simulink model "CM475A_TSG31CfgAndUse"  (R2013b)
settings: Solver=FixedStepDiscrete  SolverMode=SingleTasking  StartTime=0.0  StopTime=0.5  FixedStep=0.00005  RelTol=1e-3
undefined symbols (not defined in the file): ELECGLBPRM_PWMPERDMIN_NANOSEC_U32, sigbuilder_block, SysSt1, TSG31CfgAndUseAdcStrtOfCnvn2Offs, TSG31CfgAndUseAdcStrtOfCnvnMotCtrlPeakOffs, TSG31CfgAndUseAdcStrtOfCnvnMotCtrlVlyOffs, TSG31CfgAndUseMtrAg0SPIStart, TSG31CfgAndUsePwmDbnd, TSG31UPD_NANOSEC_U32
libraries: simulink x11, CM475A_TSG31CfgAndUse_ModelLibrary_Rev001 x11
(part 1 of 4)
settings Model: Creator=nz3zln  LastModifiedBy=nz3zln
settings SolverCC: AutoInsertRateTranBlk=on  InsertRTBMode=Always
settings DataIOCC: LimitDataPoints=off  SaveFormat=Structure  ReturnWorkspaceOutputs=on
settings OptimizationCC: BlockReduction=off  InlineParams=on  ZeroExternalMemoryAtStartup=off  ZeroInternalMemoryAtStartup=off  OptimizeModelRefInitCode=on  LifeSpan=1
settings DebuggingCC: SignalInfNanChecking=error  SignalRangeChecking=warning  UnderspecifiedInitializationDetection=Simplified  SolverPrmCheckMsg=error  InheritedTsInSrcMsg=error  DiscreteInheritContinuousMsg=error  SingleTaskRateTransMsg=error  TasksWithSamePriorityMsg=error  SigSpecEnsureSampleTimeMsg=error  CheckMatrixSingularityMsg=error  ParameterUnderflowMsg=error  ParameterPrecisionLossMsg=error  ParameterTunabilityLossMsg=error  FixptConstUnderflowMsg=warning  FixptConstOverflowMsg=warning  VectorMatrixConversionMsg=error  SignalLabelMismatchMsg=error  UnconnectedInputMsg=error  UnconnectedOutputMsg=error  UnconnectedLineMsg=error  SFcnCompatibilityMsg=error  UniqueDataStoreMsg=warning  BusObjectLabelMismatch=error  RootOutportRequireBusObject=error  AssertControl=DisableAll  ModelReferenceIOMsg=error  ModelReferenceVersionMismatchMessage=warning  ModelReferenceIOMismatchMessage=error  ModelReferenceCSMismatchMessage=warning  ModelReferenceDataLoggingMessage=error  StateNameClashWarn=warning  StrictBusMsg=ErrorOnBusTreatedAsVector  NonBusSignalsTreatedAsBus=error  SFUnexpectedBacktrackingDiag=error  SFInvalidInputDataAccessInChartInitDiag=error  SFNoUnconditionalDefaultTransitionDiag=error  SFTransitionOutsideNaturalParentDiag=error  SFUnconditionalTransitionShadowingDiag=error  SFUndirectedBroadcastEventsDiag=error
settings ModelReferenceCC: ModelReferenceNumInstancesAllowed=Single
settings RTWCC: SystemTargetFile=autosar.tlc  GenCodeOnly=on  TemplateMakefile=ert_default_tmf  Description=AUTOSAR  GenerateReport=on  ProcessScript=autosar_make_rtw_hook  LaunchReport=on
settings CodeAppCC: GenerateComments=off  IgnoreCustomStorageClasses=off  CustomSymbolStrType=$N$R$M  CustomSymbolStrBlkIO=$N$M  SimulinkBlockComments=off
settings STFCustomTargetCC: ParMdlRefBuildCompliant=on  CompOptLevelCompliant=on  IncludeMdlTerminateFcn=off  CombineOutputUpdateFcns=on  SuppressErrorStatus=on  ERTFirstTimeCompliant=on  ERTCustomFileBanners=on  SupportNonFinite=off  SupportComplex=off  SupportContinuousTime=off  SupportNonInlinedSFcns=off  MATLABClassNameForMDSCustomization=Simulink.SoftwareTarget.ERTCustomization  AutosarCompliant=on  GRTInterface=off  SystemTargetFile=autosar.tlc
settings ERTTargetCC: CodeReplacementLibrary=ANSI_C  ConcurrentExecutionCompliant=off  IncludeMdlTerminateFcn=off  SuppressErrorStatus=on  SupportNonFinite=off  SupportComplex=off  ModelStepFunctionPrototypeControlCompliant=off  CPPClassGenCompliant=off  AutosarCompliant=on  InlinedParameterPlacement=NonHierarchical  ERTCustomFileTemplate=example_file_process.tlc  EnableUserReplacementTypes=on

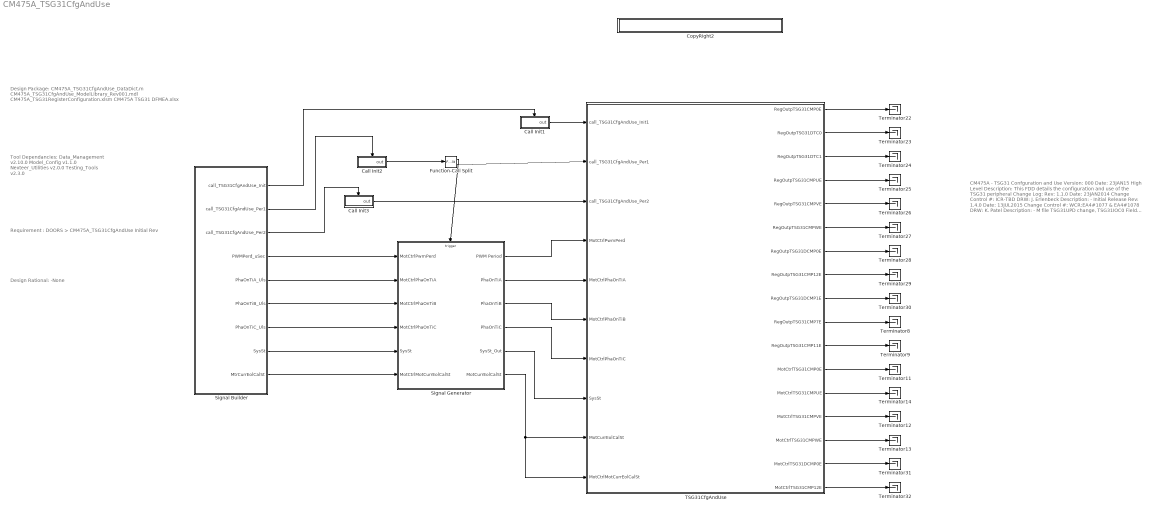
== system CM475A_TSG31CfgAndUse ==
  note: CM475A - TSG31 Confguration and Use
      |
      | Version: 000
      | Date: 23JAN15
      |
      | High Level Description:
      | This FDD details the configuration and use of the TSG31 peripheral
      |
      | Change Log:
      |
      | Rev: 1.1.0
      | Date: 23JAN2014
      | Change Control #: ICR-TBD
      | DRW: J. Erlenbeck
      | Description:
      | - Initial Release
      |
      | Rev: 1.4.0
      | Date: 13JUL2015
      | Change Control #: WCR:EA4#1077 & EA4#1078
      | DRW: K. Patel
      | Description:
      | - M file TSG31UPD change, TSG31IOC0 Field value change in excel
      |
      | Rev: 1.5.0
      | Date: 08SEP2016
      | Change Control #: WCR:EA4#7447
      | DRW: G. McCann
      | Description:
      | - M file init values changed:
      | 	MotCtrlTSG31DCMP0E
      | 	MotCtrlTSG31CMP0E
      | 	MotCtrlTSG31CMP12E
      | 	MotCtrlTSG31CMPWE
      | 	MotCtrlTSG31CMPVE
      | 	MotCtrlTSG31CMPUE
      |
      | Rev: 1.6.0
      | Date: 27SEP2016
      | Change Control #: WCR:EA4#7447
      | DRW: J. Erlenbeck
      | Description:
      | - Removed symbolic outputs, updated to newer modeling standards
      |   without changing any code functionality.
  note: Tool Dependancies:
      |
      | Data_Management v2.10.0
      | Model_Config v1.1.0
      | Nexteer_Utilities v2.0.0
      | Testing_Tools v2.3.0
  note: Design Package:
      |
      | CM475A_TSG31CfgAndUse_DataDict.m
      | CM475A_TSG31CfgAndUse_ModelLibrary_Rev001.mdl
      | CM475A_TSG31RegisterConfiguration.xlsm
      | CM475A TSG31 DFMEA.xlsx
  note: Requirement :
      |
      | DOORS > CM475A_TSG31CfgAndUse Initial Rev
  note: Design Rational:
      |
      | -None
  Call Init1 : Subsystem  TreatAsAtomicUnit=on
  Call Init2 : Subsystem  TreatAsAtomicUnit=on
  Call Init3 : Subsystem  RequirementInfo="{}  %GIDa_2aef89e2_413b_41a9_8abb_59aacf2ea464"  TreatAsAtomicUnit=on
  CopyRight2 : Subsystem  Description=|  mask(Copyright Information){none=on}
      | Copyright info block.                                               
      |                                                                     
      | Place copyright information at the top of every subsystem in design.
      mask prompts: none "No parameters"
      mask help: Place copyright information at the top of every subsystem in design.
      mask Display:
      | NxtrConf = 'Nexteer Confidential';
      | 
      | sys = bdroot; %handle for the current model ("system")
      | first = get_param(sys,'Created');
      | first = first(end-3:end);  %year is last four digits
      | 
      | last = get_param(sys,'LastModifiedDate');
      | if isempty(last)
      |     last = datestr(now,'yyyy');
      | else
      |     last = last(end-3:end);
      | end
      | 
      | if strcmp(first,last)
      |     fprintf('%s -- Copyright %s Nexteer',NxtrConf,first)
      | else
      |     fprintf('%s -- %s%s- %s Nexteer',NxtrConf,char(169),first,last)
      | end
  Function-Call Split : FunctionCallSplit
  Signal Builder : Subsystem  Tag=STV Subsys  RequirementInfo={} %GIDa_2822100e_29fa_4197_9ccc_01864625f252  LoadFcn=sigbuilder_block('load');  StartFcn=sigbuilder_block('start');  StopFcn=sigbuilder_block('stop');  ClipboardFcn=sigbuilder_block('clipboard');  mask(Sigbuilder block){}
      mask help: Simulink:masks:SigbuilderBlock_MD
      mask init:
      | if ~strcmp(get_param(bdroot(gcbh),'SimulationStatus'),'stopped') tuvar = sigbuilder_block('maskInit'); end
      settings: CopyFcn=sigbuilder_block('copy');  DeleteFcn=sigbuilder_block('delete');  ModelCloseFcn=sigbuilder_block('modelClose');  PreSaveFcn=sigbuilder_block('preSave');  PauseFcn=sigbuilder_block('pause');  ContinueFcn=sigbuilder_block('continue');  NameChangeFcn=sigbuilder_block('namechange');  OpenFcn=sigbuilder_block('open',[94.9655 670.345 1191.72 616.966 ]);  CloseFcn=sigbuilder_block('close');
      mask Display: plot(0, 0, 100, 100,[2, 2, 32, 32, 2], [68, 8, 8, 68, 68],[32, 2], [38, 38], [32, 19, 2],[53, 60, 44], [32, 17, 17, 2],[16, 16, 31, 31]);txt = getActiveGroup(gcbh);text(2, 100, txt,'verticalAlignment', 'top');
  Signal Generator : Subsystem  TreatAsAtomicUnit=on
  TSG31CfgAndUse : Subsystem
  Terminator{8..9,11..14,22..32} (17 alike) : Terminator
  wires:
  Call Init2/1(out) -> Function-Call Split/1
  Call Init3/1(out) -> TSG31CfgAndUse/3(call_TSG31CfgAndUse_Per2)
  Call Init1/1(out) -> TSG31CfgAndUse/1(call_TSG31CfgAndUse_Init1)
  Signal Builder/3(call_TSG31CfgAndUse_Per2) -> Call Init3/Enable
  Signal Builder/2(call_TSG31CfgAndUse_Per1) -> Call Init2/Enable
  Signal Builder/1(call_TSG31CfgAndUse_Init) -> Call Init1/Enable
  TSG31CfgAndUse/1(RegOutpTSG31CMP0E) -> Terminator22/1
  TSG31CfgAndUse/2(RegOutpTSG31DTC0) -> Terminator23/1
  TSG31CfgAndUse/3(RegOutpTSG31DTC1) -> Terminator24/1
  TSG31CfgAndUse/4(RegOutpTSG31CMPUE) -> Terminator25/1
  TSG31CfgAndUse/5(RegOutpTSG31CMPVE) -> Terminator26/1
  TSG31CfgAndUse/6(RegOutpTSG31CMPWE) -> Terminator27/1
  TSG31CfgAndUse/7(RegOutpTSG31DCMP0E) -> Terminator28/1
  TSG31CfgAndUse/8(RegOutpTSG31CMP12E) -> Terminator29/1
  TSG31CfgAndUse/9(RegOutpTSG31DCMP1E) -> Terminator30/1
  TSG31CfgAndUse/10(RegOutpTSG31CMP7E) -> Terminator8/1
  TSG31CfgAndUse/11(RegOutpTSG31CMP11E) -> Terminator9/1
  TSG31CfgAndUse/12(MotCtrlTSG31CMP0E) -> Terminator11/1
  TSG31CfgAndUse/13(MotCtrlTSG31CMPUE) -> Terminator14/1
  TSG31CfgAndUse/14(MotCtrlTSG31CMPVE) -> Terminator12/1
  TSG31CfgAndUse/15(MotCtrlTSG31CMPWE) -> Terminator13/1
  TSG31CfgAndUse/16(MotCtrlTSG31DCMP0E) -> Terminator31/1
  TSG31CfgAndUse/17(MotCtrlTSG31CMP12E) -> Terminator32/1
  Function-Call Split/1 -> Signal Generator/Trigger
  Function-Call Split/2 -> TSG31CfgAndUse/2(call_TSG31CfgAndUse_Per1)
  Signal Builder/7(PhaOnTiC_Uls) -> Signal Generator/4(MotCtrlPhaOnTiC)
  Signal Builder/8(SysSt) -> Signal Generator/5(SysSt)
  Signal Builder/6(PhaOnTiB_Uls) -> Signal Generator/3(MotCtrlPhaOnTiB)
  Signal Builder/5(PhaOnTiA_Uls) -> Signal Generator/2(MotCtrlPhaOnTiA)
  Signal Builder/9(MtrCurrEolCalSt) -> Signal Generator/6(MotCtrlMotCurrEolCalSt)
  Signal Builder/4(PWMPerd_uSec) -> Signal Generator/1(MotCtrlPwmPerd)
  Signal Generator/3(PhaOnTiB) -> TSG31CfgAndUse/6(MotCtrlPhaOnTiB)
  Signal Generator/2(PhaOnTiA) -> TSG31CfgAndUse/5(MotCtrlPhaOnTiA)
  Signal Generator/1(PWM Period) -> TSG31CfgAndUse/4(MotCtrlPwmPerd)
  Signal Generator/4(PhaOnTiC) -> TSG31CfgAndUse/7(MotCtrlPhaOnTiC)
  Signal Generator/5(SysSt_Out) -> TSG31CfgAndUse/8(SysSt)
  Signal Generator/6(MotCurrEolCalSt) -> TSG31CfgAndUse/10(MotCtrlMotCurrEolCalSt), TSG31CfgAndUse/9(MotCurrEolCalSt)

== system CM475A_TSG31CfgAndUse/Call Init1 ==
  Enable : EnablePort
  Function Call Trigger : simulink/Ports & Subsystems/Function-Call Generator  RequirementInfo={} %GIDa_ff755a2e_49d1_45f7_8591_3ce0ef475338  sample_time=0.002  numberOfIterations=1
  out : Outport
  wires:
  Function Call Trigger/1 -> out/1

== system CM475A_TSG31CfgAndUse/Call Init2 ==
  Enable : EnablePort
  Function Call Trigger : simulink/Ports & Subsystems/Function-Call Generator  RequirementInfo={} %GIDa_286e4ac1_b4ae_4a31_a667_8384976eef74  sample_time=0.00005  numberOfIterations=1
  out : Outport
  wires:
  Function Call Trigger/1 -> out/1

== system CM475A_TSG31CfgAndUse/Call Init3 ==
  Enable : EnablePort
  Function Call Trigger : simulink/Ports & Subsystems/Function-Call Generator  RequirementInfo={} %GIDa_f9d17251_db1b_46c2_b3b0_280e370bf339  sample_time=0.002  numberOfIterations=1
  out : Outport
  wires:
  Function Call Trigger/1 -> out/1

== system CM475A_TSG31CfgAndUse/CopyRight2 ==

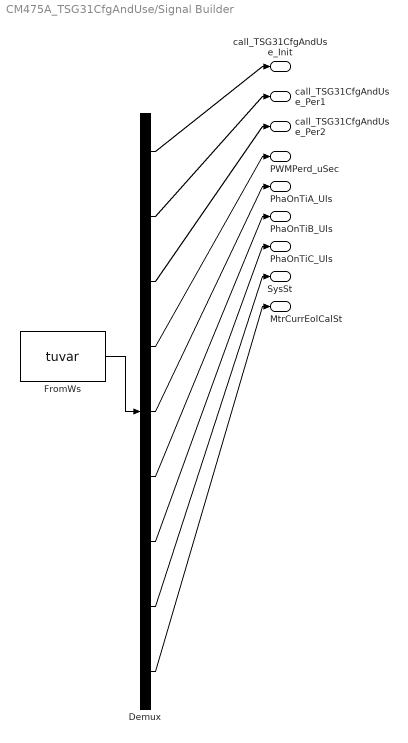
== system CM475A_TSG31CfgAndUse/Signal Builder ==
  Demux : Demux  Tag=STV Demux  Outputs=9
  FromWs : FromWorkspace  Tag=STV FromWs  VariableName=tuvar  SampleTime=0
      SigBuilderData=|
      | common.afterFinalStr = 'Extrapolate'
      | common.sampleTime = 0
      | dataSet(1).timeRange = [0 0.5]
      | dataSet(1).name = 'Group 1'
      | dataSet(2).timeRange = [0 0.5]
      | dataSet(2).name = 'Group 2'
      | dataSet(3).timeRange = [0 1.2]
      | dataSet(3).name = 'Group 3'
      | dataSet(4).timeRange = [0 5]
      | dataSet(4).name = 'Group 4'
      | dataSet(5).timeRange = [0 10]
      | dataSet(5).name = 'Group 5'
      | dataSet(6).timeRange = [0 8]
      | dataSet(6).name = 'Group 6'
      | sbobj.Groups(1).Name = 'Group 1'
      | sbobj.Groups(1).Signals(1).Name = 'call_TSG31CfgAndUse_Init'
      | sbobj.Groups(1).Signals(1).XData = [0 0.001 0.001 0.5]
      | sbobj.Groups(1).Signals(1).YData = [1 1 0 0]
      | sbobj.Groups(1).Signals(2).Name = 'call_TSG31CfgAndUse_Per1'
      | sbobj.Groups(1).Signals(2).XData = [0 0.002 0.002 0.5]
      | sbobj.Groups(1).Signals(2).YData = [0 0 1 1]
      | sbobj.Groups(1).Signals(3).Name = 'call_TSG31CfgAndUse_Per2'
      | sbobj.Groups(1).Signals(3).XData = [0 0.002 0.002 8]
      | sbobj.Groups(1).Signals(3).YData = [0 0 1 1]
      | sbobj.Groups(1).Signals(4).Name = 'PWMPerd_uSec'
      | sbobj.Groups(1).Signals(4).XData = [0 0.5]
      | sbobj.Groups(1).Signals(4).YData = [50 50]
      | sbobj.Groups(1).Signals(5).Name = 'PhaOnTiA_Uls'
      | sbobj.Groups(1).Signals(5).XData = [0 0.0102040816327 0.0204081632653 0.030612244898 0.0408163265306 0.0510204081633 0.0612244897959 0.0714285714286 0.0816326530612 0.0918367346939 0.102040816327 0.112244897959 0.122448979592 0.132653061224 0.142857142857 0.15306122449 0.163265306122 0.173469387755 0.183673469388 0.19387755102 0.204081632653 0.214285714286 0.224489795918 0.234693877551 0.244897959184 0.255102040816 0.265306122449 0.275510204082 0.285714285714 0.295918367347 0.30612244898 0.316326530612 0.326530612245 0.336734693878 0.34693877551 0.357142857143 0.367346938776 0.377551020408 0.387755102041 0.397959183673 0.408163265306 0.418367346939 0.428571428571 0.438775510204 0.448979591837 0.459183673469 0.469387755102 0.479591836735 0.489795918367 0.5]
      | sbobj.Groups(1).Signals(5).YData = [0.5 0.563938580842 0.626827291955 0.68763350244 0.745358776002 0.799055265246 0.847841275302 0.890915741234 0.927571381503 0.957206311508 0.979333926518 0.993590891707 0.9997431081 0.997689556475 0.987463956091 0.969234211025 0.943299653187 0.910086127298 0.870138998538 0.824114197654 0.772767450605 0.716941869559 0.657554109012 0.595579314351 0.53203510999 0.46796489001 0.404420685649 0.342445890988 0.283058130441 0.227232549395 0.175885802346 0.129861001462 0.0899138727015 0.0567003468135 0.0307657889751 0.0125360439091 0.0023104435254 0.000256891899656 0.00640910829277 0.0206660734817 0.0427936884921 0.0724286184973 0.109084258766 0.152158724698 0.200944734754 0.254641223998 0.31236649756 0.373172708045 0.436061419158 0.5]
      | sbobj.Groups(1).Signals(6).Name = 'PhaOnTiB_Uls'
      | sbobj.Groups(1).Signals(6).XData = [0 0.1 0.1 0.2 0.2 0.3 0.3 0.4 0.4 0.5]
      | sbobj.Groups(1).Signals(6).YData = [1 1 0 0 1 1 0 0 1 1]
      | sbobj.Groups(1).Signals(7).Name = 'PhaOnTiC_Uls'
      | sbobj.Groups(1).Signals(7).XData = [0 0.125 0.125 0.25 0.25 0.375 0.375 0.5]
      | sbobj.Groups(1).Signals(7).YData = [0 1 0 1 0 1 0 1]
      | sbobj.Groups(1).Signals(8).Name = 'SysSt'
      | sbobj.Groups(1).Signals(8).XData = [0 0 0.5 0.5 1 1 1.5 1.5 2 2 2.5 2.5 3 3 3.5 3.5 4 4 4.5 4.5 5 5 5.5 5.5 6 6 6.5 6.5 7 7 7.5 7.5 8 8]
      | sbobj.Groups(1).Signals(8).YData = [0 2 2 0 0 2 2 0 0 2 2 0 0 2 2 0 0 2 2 0 0 2 2 0 0 2 2 0 0 2 2 0 0 2]
      | sbobj.Groups(1).Signals(9).Name = 'MtrCurrEolCalSt'
      | sbobj.Groups(1).Signals(9).XData = [0 0.5 1 1 1.5 1.5 2 2 2.5 2.5 3 3 3.5 3.5 4 4 4.5 4.5 5 5 5.5 5.5 6 6 6.5 6.5 7 7 7.5 7.5 8]
      | sbobj.Groups(1).Signals(9).YData = [0 0 0 2 2 0 0 2 2 0 0 2 2 0 0 2 2 0 0 2 2 0 0 2 2 0 0 2 2 0 0]
      | sbobj.Groups(1).TimeRange = [0 0.5]
      | sbobj.Groups(2).Name = 'Group 2'
      | sbobj.Groups(2).Signals(1).Name = 'call_TSG31CfgAndUse_Init'
      | sbobj.Groups(2).Signals(1).XData = [0 0.001 0.001 0.5]
      | sbobj.Groups(2).Signals(1).YData = [1 1 0 0]
      | sbobj.Groups(2).Signals(2).Name = 'call_TSG31CfgAndUse_Per1'
      | sbobj.Groups(2).Signals(2).XData = [0 0.002 0.002 0.5]
      | sbobj.Groups(2).Signals(2).YData = [0 0 1 1]
      | sbobj.Groups(2).Signals(3).Name = 'call_TSG31CfgAndUse_Per2'
      | sbobj.Groups(2).Signals(3).XData = [0 0.002 0.002 8]
      | sbobj.Groups(2).Signals(3).YData = [0 0 1 1]
      | sbobj.Groups(2).Signals(4).Name = 'PWMPerd_uSec'
      | sbobj.Groups(2).Signals(4).XData = [0 0.5]
      | sbobj.Groups(2).Signals(4).YData = [0 0]
      | sbobj.Groups(2).Signals(5).Name = 'PhaOnTiA_Uls'
      | sbobj.Groups(2).Signals(5).XData = [0 0.5]
      | sbobj.Groups(2).Signals(5).YData = [4 4]
      | sbobj.Groups(2).Signals(6).Name = 'PhaOnTiB_Uls'
      | sbobj.Groups(2).Signals(6).XData = [0 0.2 0.2 0.5]
      | sbobj.Groups(2).Signals(6).YData = [0 0 5 5]
      | sbobj.Groups(2).Signals(7).Name = 'PhaOnTiC_Uls'
      | sbobj.Groups(2).Signals(7).XData = [0 0.5]
      | sbobj.Groups(2).Signals(7).YData = [0 0]
      | sbobj.Groups(2).Signals(8).Name = 'SysSt'
      | sbobj.Groups(2).Signals(8).XData = [0 0 0.5 0.5 1 1 1.5 1.5 2 2 2.5 2.5 3 3 3.5 3.5 4 4 4.5 4.5 5 5 5.5 5.5 6 6 6.5 6.5 7 7 7.5 7.5 8 8]
      | sbobj.Groups(2).Signals(8).YData = [0 2 2 0 0 2 2 0 0 2 2 0 0 2 2 0 0 2 2 0 0 2 2 0 0 2 2 0 0 2 2 0 0 2]
      | sbobj.Groups(2).Signals(9).Name = 'MtrCurrEolCalSt'
      | sbobj.Groups(2).Signals(9).XData = [0 0 0.5 0.5 1 1 1.5 1.5 2 2 2.5 2.5 3 3 3.5 3.5 4 4 4.5 4.5 5 5 5.5 5.5 6 6 6.5 6.5 7 7 7.5 7.5 8 8]
      | sbobj.Groups(2).Signals(9).YData = [0 2 2 0 0 2 2 0 0 2 2 0 0 2 2 0 0 2 2 0 0 2 2 0 0 2 2 0 0 2 2 0 0 2]
      | sbobj.Groups(2).TimeRange = [0 0.5]
      | sbobj.Groups(3).Name = 'Group 3'
      | sbobj.Groups(3).Signals(1).Name = 'call_TSG31CfgAndUse_Init'
      | sbobj.Groups(3).Signals(1).XData = [0 0.001 0.001 1.2]
      | sbobj.Groups(3).Signals(1).YData = [1 1 0 0]
      | sbobj.Groups(3).Signals(2).Name = 'call_TSG31CfgAndUse_Per1'
      | sbobj.Groups(3).Signals(2).XData = [0 0.002 0.002 1.2]
      | sbobj.Groups(3).Signals(2).YData = [0 0 1 1]
      | sbobj.Groups(3).Signals(3).Name = 'call_TSG31CfgAndUse_Per2'
      | sbobj.Groups(3).Signals(3).XData = [0 0.002 0.002 8]
      | sbobj.Groups(3).Signals(3).YData = [0 0 1 1]
      | sbobj.Groups(3).Signals(4).Name = 'PWMPerd_uSec'
      | sbobj.Groups(3).Signals(4).XData = [0 1.2]
      | sbobj.Groups(3).Signals(4).YData = [0 0]
      | sbobj.Groups(3).Signals(5).Name = 'PhaOnTiA_Uls'
      | sbobj.Groups(3).Signals(5).XData = [0 1 1 1.2]
      | sbobj.Groups(3).Signals(5).YData = [0 0 -5 -5]
      | sbobj.Groups(3).Signals(6).Name = 'PhaOnTiB_Uls'
      | sbobj.Groups(3).Signals(6).XData = [0 1.2]
      | sbobj.Groups(3).Signals(6).YData = [0.5 0.5]
      | sbobj.Groups(3).Signals(7).Name = 'PhaOnTiC_Uls'
      | sbobj.Groups(3).Signals(7).XData = [0 1.2]
      | sbobj.Groups(3).Signals(7).YData = [0 0]
      | sbobj.Groups(3).Signals(8).Name = 'SysSt'
      | sbobj.Groups(3).Signals(8).XData = [0 0 0.5 0.5 1 1 1.5 1.5 2 2 2.5 2.5 3 3 3.5 3.5 4 4 4.5 4.5 5 5 5.5 5.5 6 6 6.5 6.5 7 7 7.5 7.5 8 8]
      | sbobj.Groups(3).Signals(8).YData = [0 2 2 0 0 2 2 0 0 2 2 0 0 2 2 0 0 2 2 0 0 2 2 0 0 2 2 0 0 2 2 0 0 2]
      | sbobj.Groups(3).Signals(9).Name = 'MtrCurrEolCalSt'
      | sbobj.Groups(3).Signals(9).XData = [0 0 0.5 0.5 1 1 1.5 1.5 2 2 2.5 2.5 3 3 3.5 3.5 4 4 4.5 4.5 5 5 5.5 5.5 6 6 6.5 6.5 7 7 7.5 7.5 8 8]
      | sbobj.Groups(3).Signals(9).YData = [0 2 2 0 0 2 2 0 0 2 2 0 0 2 2 0 0 2 2 0 0 2 2 0 0 2 2 0 0 2 2 0 0 2]
      | sbobj.Groups(3).TimeRange = [0 1.2]
      | sbobj.Groups(4).Name = 'Group 4'
      | sbobj.Groups(4).Signals(1).Name = 'call_TSG31CfgAndUse_Init'
      | sbobj.Groups(4).Signals(1).XData = [0 0.001 0.001 5]
      | sbobj.Groups(4).Signals(1).YData = [1 1 0 0]
      | sbobj.Groups(4).Signals(2).Name = 'call_TSG31CfgAndUse_Per1'
      | sbobj.Groups(4).Signals(2).XData = [0 0.002 0.002 5]
      | sbobj.Groups(4).Signals(2).YData = [0 0 1 1]
      | sbobj.Groups(4).Signals(3).Name = 'call_TSG31CfgAndUse_Per2'
      | sbobj.Groups(4).Signals(3).XData = [0 0.002 0.002 8]
      | sbobj.Groups(4).Signals(3).YData = [0 0 1 1]
      | sbobj.Groups(4).Signals(4).Name = 'PWMPerd_uSec'
      | sbobj.Groups(4).Signals(4).XData = [0 5]
      | sbobj.Groups(4).Signals(4).YData = [0 0]
      | sbobj.Groups(4).Signals(5).Name = 'PhaOnTiA_Uls'
      | sbobj.Groups(4).Signals(5).XData = [0 1.5 2 5]
      | sbobj.Groups(4).Signals(5).YData = [0 1.35 0.6 -3]
      | sbobj.Groups(4).Signals(6).Name = 'PhaOnTiB_Uls'
      | sbobj.Groups(4).Signals(6).XData = [0 0.1 0.1 5]
      | sbobj.Groups(4).Signals(6).YData = [0 0 2 2]
      | sbobj.Groups(4).Signals(7).Name = 'PhaOnTiC_Uls'
      | sbobj.Groups(4).Signals(7).XData = [0 5]
      | sbobj.Groups(4).Signals(7).YData = [0 0]
      | sbobj.Groups(4).Signals(8).Name = 'SysSt'
      | sbobj.Groups(4).Signals(8).XData = [0 0 0.5 0.5 1 1 1.5 1.5 2 2 2.5 2.5 3 3 3.5 3.5 4 4 4.5 4.5 5 5 5.5 5.5 6 6 6.5 6.5 7 7 7.5 7.5 8 8]
      | sbobj.Groups(4).Signals(8).YData = [0 2 2 0 0 2 2 0 0 2 2 0 0 2 2 0 0 2 2 0 0 2 2 0 0 2 2 0 0 2 2 0 0 2]
      | sbobj.Groups(4).Signals(9).Name = 'MtrCurrEolCalSt'
      | sbobj.Groups(4).Signals(9).XData = [0 0 0.5 0.5 1 1 1.5 1.5 2 2 2.5 2.5 3 3 3.5 3.5 4 4 4.5 4.5 5 5 5.5 5.5 6 6 6.5 6.5 7 7 7.5 7.5 8 8]
      | sbobj.Groups(4).Signals(9).YData = [0 2 2 0 0 2 2 0 0 2 2 0 0 2 2 0 0 2 2 0 0 2 2 0 0 2 2 0 0 2 2 0 0 2]
      | sbobj.Groups(4).TimeRange = [0 5]
      | sbobj.Groups(5).Name = 'Group 5'
      | sbobj.Groups(5).Signals(1).Name = 'call_TSG31CfgAndUse_Init'
      | sbobj.Groups(5).Signals(1).XData = [0 0.001 0.001 10]
      | sbobj.Groups(5).Signals(1).YData = [1 1 0 0]
      | sbobj.Groups(5).Signals(2).Name = 'call_TSG31CfgAndUse_Per1'
      | sbobj.Groups(5).Signals(2).XData = [0 0.002 0.002 10]
      | sbobj.Groups(5).Signals(2).YData = [0 0 1 1]
      | sbobj.Groups(5).Signals(3).Name = 'call_TSG31CfgAndUse_Per2'
      | sbobj.Groups(5).Signals(3).XData = [0 0.002 0.002 10]
      | sbobj.Groups(5).Signals(3).YData = [0 0 1 1]
      | sbobj.Groups(5).Signals(4).Name = 'PWMPerd_uSec'
      | sbobj.Groups(5).Signals(4).XData = [0 10]
      | sbobj.Groups(5).Signals(4).YData = [0 0]
      | sbobj.Groups(5).Signals(5).Name = 'PhaOnTiA_Uls'
      | sbobj.Groups(5).Signals(5).XData = [0 10]
      | sbobj.Groups(5).Signals(5).YData = [2 2]
      | sbobj.Groups(5).Signals(6).Name = 'PhaOnTiB_Uls'
      | sbobj.Groups(5).Signals(6).XData = [0 10]
      | sbobj.Groups(5).Signals(6).YData = [2.5 2.5]
      | sbobj.Groups(5).Signals(7).Name = 'PhaOnTiC_Uls'
      | sbobj.Groups(5).Signals(7).XData = [0 4 5 10]
      | sbobj.Groups(5).Signals(7).YData = [0 59 70 511]
      | sbobj.Groups(5).Signals(8).Name = 'SysSt'
      | sbobj.Groups(5).Signals(8).XData = [0 0 0.5 0.5 1 1 1.5 1.5 2 2 2.5 2.5 3 3 3.5 3.5 4 4 4.5 4.5 5 5 5.5 5.5 6 6 6.5 6.5 7 7 7.5 7.5 8 8 10]
      | sbobj.Groups(5).Signals(8).YData = [0 2 2 0 0 2 2 0 0 2 2 0 0 2 2 0 0 2 2 0 0 2 2 0 0 2 2 0 0 2 2 0 0 2 2]
      | sbobj.Groups(5).Signals(9).Name = 'MtrCurrEolCalSt'
      | sbobj.Groups(5).Signals(9).XData = [0 0 0.5 0.5 1 1 1.5 1.5 2 2 2.5 2.5 3 3 3.5 3.5 4 4 4.5 4.5 5 5 5.5 5.5 6 6 6.5 6.5 7 7 7.5 7.5 8 8 10]
      | sbobj.Groups(5).Signals(9).YData = [0 2 2 0 0 2 2 0 0 2 2 0 0 2 2 0 0 2 2 0 0 2 2 0 0 2 2 0 0 2 2 0 0 2 2]
      | sbobj.Groups(6).Name = 'Group 6'
      | sbobj.Groups(6).Signals(1).Name = 'call_TSG31CfgAndUse_Init'
      | sbobj.Groups(6).Signals(1).XData = [0 0.001 0.001 8]
      | sbobj.Groups(6).Signals(1).YData = [1 1 0 0]
      | sbobj.Groups(6).Signals(2).Name = 'call_TSG31CfgAndUse_Per1'
      | sbobj.Groups(6).Signals(2).XData = [0 0.002 0.002 8]
      | sbobj.Groups(6).Signals(2).YData = [0 0 1 1]
      | sbobj.Groups(6).Signals(3).Name = 'call_TSG31CfgAndUse_Per2'
      | sbobj.Groups(6).Signals(3).XData = [0 0.002 0.002 8]
      | sbobj.Groups(6).Signals(3).YData = [0 0 1 1]
      | sbobj.Groups(6).Signals(4).Name = 'PWMPerd_uSec'
      | sbobj.Groups(6).Signals(4).XData = [0 0.125 0.25 0.375 0.5 0.625 0.75 0.875 1 1.125 1.25 1.375 1.5 1.625 1.75 1.875 2 2.125 2.25 2.375 2.5 2.625 2.75 2.875 3 3.125 3.25 3.375 3.5 3.625 3.75 3.875 4 4.125 4.25 4.375 4.5 4.625 4.75 4.875 5 5.125 5.25 5.375 5.5 5.625 5.75 5.875 6 6.125 6.25 6.375 6.5 6.625 6.75 6.875 7 7.125 7.25 7.375 7.5 7.625 7.75 7.875 8]
      | sbobj.Groups(6).Signals(4).YData = [1 1.70710678119 2 1.70710678119 1 0.292893218813 0 0.292893218813 1 1.70710678119 2 1.70710678119 1 0.292893218813 0 0.292893218813 1 1.70710678119 2 1.70710678119 1 0.292893218813 0 0.292893218813 1 1.70710678119 2 1.70710678119 1 0.292893218813 0 0.292893218813 1 1.70710678119 2 1.70710678119 1 0.292893218813 0 0.292893218813 1 1.70710678119 2 1.70710678119 1 0.292893218813 0 0.292893218813 1 1.70710678119 2 1.70710678119 1 0.292893218813 0 0.292893218813 1 1.70710678119 2 1.70710678119 1 0.292893218813 0 0.292893218813 1]
      | sbobj.Groups(6).Signals(5).Name = 'PhaOnTiA_Uls'
      | sbobj.Groups(6).Signals(5).XData = [0 0.5 0.5 1 1 1.5 1.5 2 2 2.5 2.5 3 3 3.5 3.5 4 4 4.5 5 5.5 6 6.5 6.5 7 7.5 7.5 8]
      | sbobj.Groups(6).Signals(5).YData = [10 10 -10 -10 10 10 -10 -10 10 10 -10 -10 7 5.5 -5 -5.5 0 0 0 0 0 0 -0.5 0 -0.5 0 0]
      | sbobj.Groups(6).Signals(6).Name = 'PhaOnTiB_Uls'
      | sbobj.Groups(6).Signals(6).XData = [0 1 1 2 2 3 3 4 4 5 5 6 6 7 7 8]
      | sbobj.Groups(6).Signals(6).YData = [8.8 8.8 -8.8 -8.8 8.8 8.8 -8.8 -8.8 8.8 8.8 -8.8 -8.8 8.8 8.8 -8.8 -8.6]
      | sbobj.Groups(6).Signals(7).Name = 'PhaOnTiC_Uls'
      | sbobj.Groups(6).Signals(7).XData = [0 8]
      | sbobj.Groups(6).Signals(7).YData = [70 70]
      | sbobj.Groups(6).Signals(8).Name = 'SysSt'
      | sbobj.Groups(6).Signals(8).XData = [0 0.5 0.5 1 1 1.5 1.5 2 2 2.5 2.5 3 3 3.5 3.5 4 4 4.5 4.5 5 5 5.5 5.5 6 6 6.5 6.5 7 7 7.5 7.5 8]
      | sbobj.Groups(6).Signals(8).YData = [2 2 0 0 2 2 0 0 2 2 0 0 2 2 0 0 2 2 0 0 2 2 0 0 2 2 0 0 2 2 0 0]
      | sbobj.Groups(6).Signals(9).Name = 'MtrCurrEolCalSt'
      | sbobj.Groups(6).Signals(9).XData = [0 0.5 0.5 1 1 1.5 1.5 2 2 2.5 2.5 3 3 3.5 3.5 4 4 4.5 4.5 5 5 5.5 5.5 6 6 6.5 6.5 7 7 7.5 7.5 8]
      | sbobj.Groups(6).Signals(9).YData = [2 2 0 0 2 2 0 0 2 2 0 0 2 2 0 0 2 2 0 0 2 2 0 0 2 2 0 0 2 2 0 0]
      | sbobj.Groups(6).TimeRange = [0 8]
  call_TSG31CfgAndUse_Init : Outport  Tag=STV Outport
  call_TSG31CfgAndUse_Per1 : Outport  Tag=STV Outport  Port=2
  call_TSG31CfgAndUse_Per2 : Outport  Tag=STV Outport  Port=3
  PWMPerd_uSec : Outport  Tag=STV Outport  Port=4
  PhaOnTiA_Uls : Outport  Tag=STV Outport  Port=5
  PhaOnTiB_Uls : Outport  Tag=STV Outport  Port=6
  PhaOnTiC_Uls : Outport  Tag=STV Outport  Port=7
  SysSt : Outport  Tag=STV Outport  Port=8
  MtrCurrEolCalSt : Outport  Tag=STV Outport  Port=9
  wires:
  FromWs/1 -> Demux/1
  Demux/1 -> call_TSG31CfgAndUse_Init/1
  Demux/2 -> call_TSG31CfgAndUse_Per1/1
  Demux/3 -> call_TSG31CfgAndUse_Per2/1
  Demux/4 -> PWMPerd_uSec/1
  Demux/5 -> PhaOnTiA_Uls/1
  Demux/6 -> PhaOnTiB_Uls/1
  Demux/7 -> PhaOnTiC_Uls/1
  Demux/8 -> SysSt/1
  Demux/9 -> MtrCurrEolCalSt/1

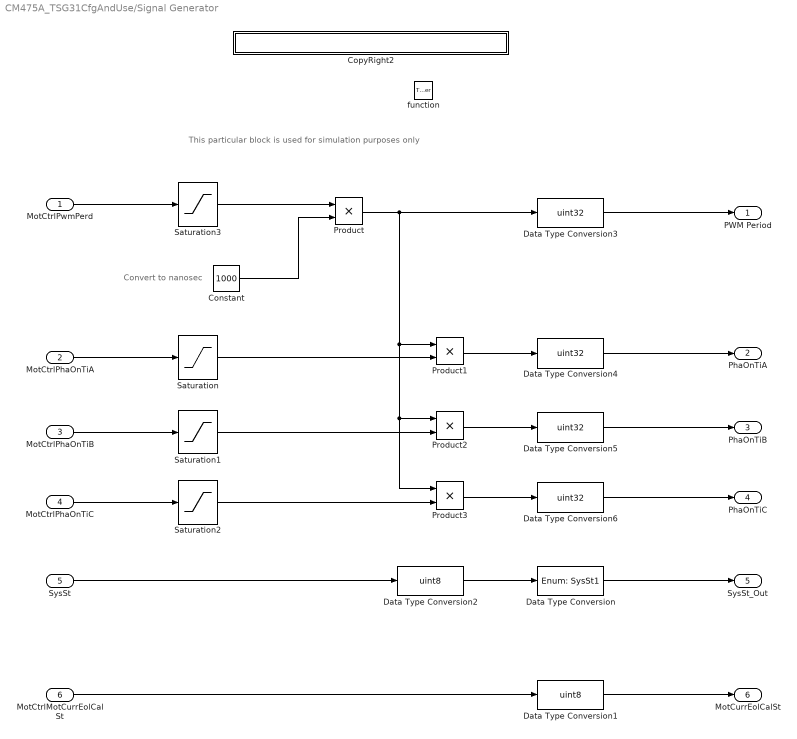
== system CM475A_TSG31CfgAndUse/Signal Generator ==
  note: Convert to nanosec
  note: This particular block is used for simulation purposes only
  MotCtrlPwmPerd : Inport
  MotCtrlPhaOnTiA : Inport  Port=2
  MotCtrlPhaOnTiB : Inport  Port=3
  MotCtrlPhaOnTiC : Inport  Port=4
  SysSt : Inport  RequirementInfo={'linktype_rmi_doors' '000089b8 (/ESG Group/FDD Module Requirements/ES FDDs/CM475A - TSG31 Configuration and Use)' '#CM475A_86' 'true' 'REQ: CM475A_86' '' } %GIDa_7649ba70_f370_4d93_9448_0ee2e543fc9b  Port=5
  MotCtrlMotCurrEolCalSt : Inport  Port=6
  function : TriggerPort  TriggerType=function-call
  Constant : Constant  Value=1000
  CopyRight2 : Subsystem  Description=|  mask(Copyright Information){none=on}
      | Copyright info block.                                               
      |                                                                     
      | Place copyright information at the top of every subsystem in design.
      mask prompts: none "No parameters"
      mask help: Place copyright information at the top of every subsystem in design.
      mask Display:
      | NxtrConf = 'Nexteer Confidential';
      | 
      | sys = bdroot; %handle for the current model ("system")
      | first = get_param(sys,'Created');
      | first = first(end-3:end);  %year is last four digits
      | 
      | last = get_param(sys,'LastModifiedDate');
      | if isempty(last)
      |     last = datestr(now,'yyyy');
      | else
      |     last = last(end-3:end);
      | end
      | 
      | if strcmp(first,last)
      |     fprintf('%s -- Copyright %s Nexteer',NxtrConf,first)
      | else
      |     fprintf('%s -- %s%s- %s Nexteer',NxtrConf,char(169),first,last)
      | end
  Data Type Conversion : DataTypeConversion  OutDataTypeStr=Enum: SysSt1
  Data Type Conversion1 : DataTypeConversion  OutDataTypeStr=uint8
  Data Type Conversion2 : DataTypeConversion  OutDataTypeStr=uint8
  Data Type Conversion{3..6} (4 alike) : DataTypeConversion  OutDataTypeStr=uint32
  Product{,1..3} (4 alike) : Product
  Saturation : Saturate  UpperLimit=1  LowerLimit=0
  Saturation1 : Saturate  UpperLimit=1  LowerLimit=0
  Saturation2 : Saturate  UpperLimit=1  LowerLimit=0
  Saturation3 : Saturate  UpperLimit=1e6/14e3  LowerLimit=1e6/22e3
  PWM Period : Outport
  PhaOnTiA : Outport  Port=2
  PhaOnTiB : Outport  Port=3
  PhaOnTiC : Outport  Port=4
  SysSt_Out : Outport  Port=5
  MotCurrEolCalSt : Outport  Port=6
  wires:
  Data Type Conversion2/1 -> Data Type Conversion/1
  SysSt/1 -> Data Type Conversion2/1
  MotCtrlMotCurrEolCalSt/1 -> Data Type Conversion1/1
  MotCtrlPhaOnTiA/1 -> Saturation/1
  MotCtrlPhaOnTiB/1 -> Saturation1/1
  MotCtrlPhaOnTiC/1 -> Saturation2/1
  MotCtrlPwmPerd/1 -> Saturation3/1
  Saturation3/1 -> Product/1
  Constant/1 -> Product/2
  Product/1 -> Data Type Conversion3/1, Product3/1, Product2/1, Product1/1
  Saturation/1 -> Product1/2
  Saturation1/1 -> Product2/2
  Saturation2/1 -> Product3/2
  Product1/1 -> Data Type Conversion4/1
  Product2/1 -> Data Type Conversion5/1
  Product3/1 -> Data Type Conversion6/1
  Data Type Conversion3/1 -> PWM Period/1
  Data Type Conversion4/1 -> PhaOnTiA/1
  Data Type Conversion5/1 -> PhaOnTiB/1
  Data Type Conversion6/1 -> PhaOnTiC/1
  Data Type Conversion1/1 -> MotCurrEolCalSt/1
  Data Type Conversion/1 -> SysSt_Out/1

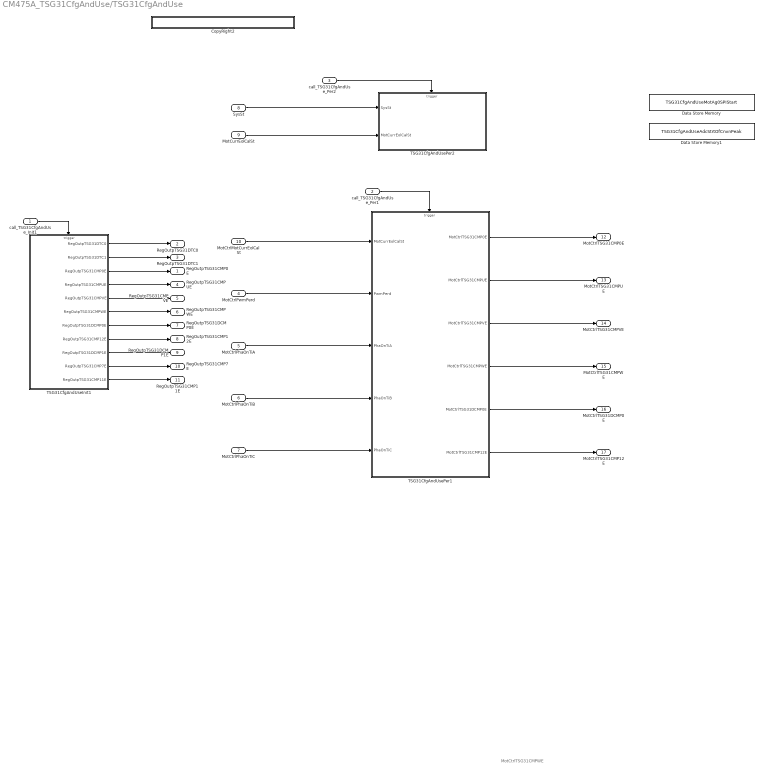
== system CM475A_TSG31CfgAndUse/TSG31CfgAndUse ==
  note: MotCtrlTSG31CMPWE
  call_TSG31CfgAndUse_Init1 : Inport
  call_TSG31CfgAndUse_Per1 : Inport  Port=2
  call_TSG31CfgAndUse_Per2 : Inport  Port=3
  MotCtrlPwmPerd : Inport  Port=4
  MotCtrlPhaOnTiA : Inport  Port=5
  MotCtrlPhaOnTiB : Inport  Port=6
  MotCtrlPhaOnTiC : Inport  Port=7
  SysSt : Inport  RequirementInfo={'linktype_rmi_doors' '000089b8 (/ESG Group/FDD Module Requirements/ES FDDs/CM475A - TSG31 Configuration and Use)' '#CM475A_86' 'true' 'REQ: CM475A_86' '' } %GIDa_aa8546c3_6590_4ff0_9f9c_9dfa76e6fbbf  Port=8  OutDataTypeStr=Enum: SysSt1
  MotCurrEolCalSt : Inport  Port=9  OutDataTypeStr=uint8
  MotCtrlMotCurrEolCalSt : Inport  Port=10  OutDataTypeStr=uint8
  CopyRight2 : Subsystem  Description=|  mask(Copyright Information){none=on}
      | Copyright info block.                                               
      |                                                                     
      | Place copyright information at the top of every subsystem in design.
      mask prompts: none "No parameters"
      mask help: Place copyright information at the top of every subsystem in design.
      mask Display:
      | NxtrConf = 'Nexteer Confidential';
      | 
      | sys = bdroot; %handle for the current model ("system")
      | first = get_param(sys,'Created');
      | first = first(end-3:end);  %year is last four digits
      | 
      | last = get_param(sys,'LastModifiedDate');
      | if isempty(last)
      |     last = datestr(now,'yyyy');
      | else
      |     last = last(end-3:end);
      | end
      | 
      | if strcmp(first,last)
      |     fprintf('%s -- Copyright %s Nexteer',NxtrConf,first)
      | else
      |     fprintf('%s -- %s%s- %s Nexteer',NxtrConf,char(169),first,last)
      | end
  Data Store Memory : DataStoreMemory  DataStoreName=TSG31CfgAndUseMotAg0SPIStart  StateMustResolveToSignalObject=on
  Data Store Memory1 : DataStoreMemory  DataStoreName=TSG31CfgAndUseAdcStrtOfCnvnPeak  StateMustResolveToSignalObject=on
  TSG31CfgAndUseInit1 : Subsystem
  TSG31CfgAndUsePer1 : Subsystem
  TSG31CfgAndUsePer2 : Subsystem  RequirementInfo={'linktype_rmi_doors' '000089b8 (/ESG Group/FDD Module Requirements/ES FDDs/CM475A - TSG31 Configuration and Use)' '#CM475A_15' 'true' 'REQ: CM475A_15' '' ; 'linktype_rmi_doors' '000089b8 (/ESG Group/FDD Module Requirements/ES FDDs/CM475A - TSG31 Configuration and Use)' '#CM475A_71' 'true' 'REQ: CM475A_71' '' ; 'linktype_rmi_doors' '000089b8 (/ESG Group/FDD Module Requirements/ES FDDs/CM475A - TSG31 Configuration and Use)' '#CM475A_70' 'true' 'REQ: CM475A_70' '' ; 'linktype_rmi_doors' '000089b8 (/ESG Group/FDD Module Requirements/ES FDDs/CM475A - TSG31 Configuration and Use)' '#CM475A_69' 'true' 'REQ: CM475A_69' '' ; 'linktype_rmi_doors' '000089b8 (/ESG Group/FDD Module Requirements/ES FDDs/CM475A - TSG31 Configuration and Use)' '#CM475A_68' 'true' 'REQ: CM475A_68' '' ; 'linktype_rmi_doors' '000089b8 (/ESG Group/FDD Module Requirements/ES FDDs/CM475A - TSG31 Configuration and Use)' '#CM475A_67' 'true' 'REQ: CM475A_67' '' } %GIDa_629aaa7a_78eb_449a_8685_c96cc51ef040
  RegOutpTSG31CMP0E : Outport  RequirementInfo={'linktype_rmi_doors' '000089b8 (/ESG Group/FDD Module Requirements/ES FDDs/CM475A - TSG31 Configuration and Use)' '#CM475A_80' 'true' 'REQ: CM475A_80' '' } %GIDa_a5a4cad5_b101_4d73_a2f9_d825a0fe7ad1
  RegOutpTSG31DTC0 : Outport  Port=2
  RegOutpTSG31DTC1 : Outport  Port=3
  RegOutpTSG31CMPUE : Outport  Port=4
  RegOutpTSG31CMPVE : Outport  Port=5
  RegOutpTSG31CMPWE : Outport  Port=6
  RegOutpTSG31DCMP0E : Outport  Port=7
  RegOutpTSG31CMP12E : Outport  Port=8
  RegOutpTSG31DCMP1E : Outport  Port=9
  RegOutpTSG31CMP7E : Outport  Port=10
  RegOutpTSG31CMP11E : Outport  Port=11
  MotCtrlTSG31CMP0E : Outport  Port=12
  MotCtrlTSG31CMPUE : Outport  Port=13
  MotCtrlTSG31CMPVE : Outport  Port=14
  MotCtrlTSG31CMPWE : Outport  Port=15
  MotCtrlTSG31DCMP0E : Outport  Port=16
  MotCtrlTSG31CMP12E : Outport  Port=17
  wires:
  MotCtrlPhaOnTiA/1 -> TSG31CfgAndUsePer1/3(PhaOnTiA)
  MotCtrlPhaOnTiB/1 -> TSG31CfgAndUsePer1/4(PhaOnTiB)
  MotCtrlPhaOnTiC/1 -> TSG31CfgAndUsePer1/5(PhaOnTiC)
  SysSt/1 -> TSG31CfgAndUsePer2/1(SysSt)
  MotCtrlPwmPerd/1 -> TSG31CfgAndUsePer1/2(PwmPerd)
  call_TSG31CfgAndUse_Init1/1 -> TSG31CfgAndUseInit1/Trigger
  call_TSG31CfgAndUse_Per1/1 -> TSG31CfgAndUsePer1/Trigger
  call_TSG31CfgAndUse_Per2/1 -> TSG31CfgAndUsePer2/Trigger
  MotCurrEolCalSt/1 -> TSG31CfgAndUsePer2/2(MotCurrEolCalSt)
  TSG31CfgAndUseInit1/1(RegOutpTSG31DTC0) -> RegOutpTSG31DTC0/1
  TSG31CfgAndUseInit1/2(RegOutpTSG31DTC1) -> RegOutpTSG31DTC1/1
  TSG31CfgAndUseInit1/3(RegOutpTSG31CMP0E) -> RegOutpTSG31CMP0E/1
  TSG31CfgAndUseInit1/4(RegOutpTSG31CMPUE) -> RegOutpTSG31CMPUE/1
  TSG31CfgAndUseInit1/5(RegOutpTSG31CMPVE) -> RegOutpTSG31CMPVE/1
  TSG31CfgAndUseInit1/6(RegOutpTSG31CMPWE) -> RegOutpTSG31CMPWE/1
  TSG31CfgAndUseInit1/7(RegOutpTSG31DCMP0E) -> RegOutpTSG31DCMP0E/1
  TSG31CfgAndUseInit1/8(RegOutpTSG31CMP12E) -> RegOutpTSG31CMP12E/1
  TSG31CfgAndUseInit1/9(RegOutpTSG31DCMP1E) -> RegOutpTSG31DCMP1E/1
  TSG31CfgAndUseInit1/10(RegOutpTSG31CMP7E) -> RegOutpTSG31CMP7E/1
  TSG31CfgAndUseInit1/11(RegOutpTSG31CMP11E) -> RegOutpTSG31CMP11E/1
  MotCtrlMotCurrEolCalSt/1 -> TSG31CfgAndUsePer1/1(MotCurrEolCalSt)
  TSG31CfgAndUsePer1/2(MotCtrlTSG31CMPUE) -> MotCtrlTSG31CMPUE/1
  TSG31CfgAndUsePer1/3(MotCtrlTSG31CMPVE) -> MotCtrlTSG31CMPVE/1
  TSG31CfgAndUsePer1/4(MotCtrlTSG31CMPWE) -> MotCtrlTSG31CMPWE/1
  TSG31CfgAndUsePer1/1(MotCtrlTSG31CMP0E) -> MotCtrlTSG31CMP0E/1
  TSG31CfgAndUsePer1/5(MotCtrlTSG31DCMP0E) -> MotCtrlTSG31DCMP0E/1
  TSG31CfgAndUsePer1/6(MotCtrlTSG31CMP12E) -> MotCtrlTSG31CMP12E/1

== system CM475A_TSG31CfgAndUse/Signal Generator/CopyRight2 ==

== system CM475A_TSG31CfgAndUse/TSG31CfgAndUse/CopyRight2 ==

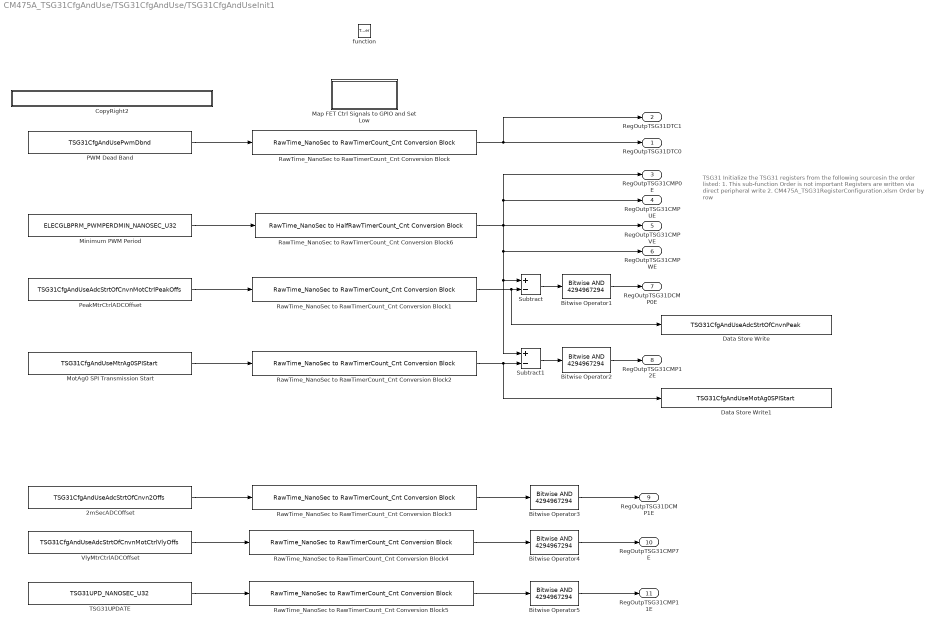
== system CM475A_TSG31CfgAndUse/TSG31CfgAndUse/TSG31CfgAndUseInit1 ==
  note: TSG31
      | Initialize the TSG31 registers from the following sourcesin the order listed:
      | 1. This sub-function
      |     Order is not important
      |     Registers are written via direct peripheral write
      | 2. CM475A_TSG31RegisterConfiguration.xlsm
      |     Order by row
  function : TriggerPort  TriggerType=function-call
  2mSecADCOffset : Constant  Value=TSG31CfgAndUseAdcStrtOfCnvn2Offs  OutDataTypeStr=uint32
  Bitwise Operator{1..5} (5 alike) : simulink/Logic and Bit Operations/Bitwise Operator  logicop=AND  UseBitMask=on  BitMask=4294967294  BitMaskRealWorld=Stored Integer
  CopyRight2 : Subsystem  Description=|  mask(Copyright Information){none=on}
      | Copyright info block.                                               
      |                                                                     
      | Place copyright information at the top of every subsystem in design.
      mask prompts: none "No parameters"
      mask help: Place copyright information at the top of every subsystem in design.
      mask Display:
      | NxtrConf = 'Nexteer Confidential';
      | 
      | sys = bdroot; %handle for the current model ("system")
      | first = get_param(sys,'Created');
      | first = first(end-3:end);  %year is last four digits
      | 
      | last = get_param(sys,'LastModifiedDate');
      | if isempty(last)
      |     last = datestr(now,'yyyy');
      | else
      |     last = last(end-3:end);
      | end
      | 
      | if strcmp(first,last)
      |     fprintf('%s -- Copyright %s Nexteer',NxtrConf,first)
      | else
      |     fprintf('%s -- %s%s- %s Nexteer',NxtrConf,char(169),first,last)
      | end
  Data Store Write : DataStoreWrite  DataStoreName=TSG31CfgAndUseAdcStrtOfCnvnPeak
  Data Store Write1 : DataStoreWrite  DataStoreName=TSG31CfgAndUseMotAg0SPIStart
  Map FET Ctrl Signals to GPIO and Set Low : Subsystem  RequirementInfo={'linktype_rmi_doors' '000089b8 (/ESG Group/FDD Module Requirements/ES FDDs/CM475A - TSG31 Configuration and Use)' '#CM475A_15' 'true' 'REQ: CM475A_15' '' ; 'linktype_rmi_doors' '000089b8 (/ESG Group/FDD Module Requirements/ES FDDs/CM475A - TSG31 Configuration and Use)' '#CM475A_71' 'true' 'REQ: CM475A_71' '' ; 'linktype_rmi_doors' '000089b8 (/ESG Group/FDD Module Requirements/ES FDDs/CM475A - TSG31 Configuration and Use)' '#CM475A_70' 'true' 'REQ: CM475A_70' '' ; 'linktype_rmi_doors' '000089b8 (/ESG Group/FDD Module Requirements/ES FDDs/CM475A - TSG31 Configuration and Use)' '#CM475A_69' 'true' 'REQ: CM475A_69' '' ; 'linktype_rmi_doors' '000089b8 (/ESG Group/FDD Module Requirements/ES FDDs/CM475A - TSG31 Configuration and Use)' '#CM475A_68' 'true' 'REQ: CM475A_68' '' ; 'linktype_rmi_doors' '000089b8 (/ESG Group/FDD Module Requirements/ES FDDs/CM475A - TSG31 Configuration and Use)' '#CM475A_67' 'true' 'REQ: CM475A_67' '' } %GIDa_f23f8d09_839d_4171_80cd_77ba6fbd0169
  Minimum PWM Period : Constant  Value=ELECGLBPRM_PWMPERDMIN_NANOSEC_U32  OutDataTypeStr=uint32
  MotAg0 SPI Transmission Start : Constant  Value=TSG31CfgAndUseMtrAg0SPIStart  OutDataTypeStr=uint32
  PWM Dead Band : Constant  Value=TSG31CfgAndUsePwmDbnd  OutDataTypeStr=uint32
  PeakMtrCtrlADCOffset : Constant  Value=TSG31CfgAndUseAdcStrtOfCnvnMotCtrlPeakOffs  OutDataTypeStr=uint32
  RawTime_NanoSec to RawTimerCount_Cnt Conversion Block{,1..5} (6 alike) : CM475A_TSG31CfgAndUse_ModelLibrary_Rev001/RawTime_NanoSec to RawTimerCount_Cnt Conversion Block
  RawTime_NanoSec to RawTimerCount_Cnt Conversion Block6 : CM475A_TSG31CfgAndUse_ModelLibrary_Rev001/RawTime_NanoSec to HalfRawTimerCount_Cnt Conversion Block
  Subtract : Sum  Inputs=+-
  Subtract1 : Sum  Inputs=+-
  TSG31UPDATE : Constant  Value=TSG31UPD_NANOSEC_U32  OutDataTypeStr=uint32
  VlyMtrCtrlADCOffset : Constant  Value=TSG31CfgAndUseAdcStrtOfCnvnMotCtrlVlyOffs  OutDataTypeStr=uint32
  RegOutpTSG31DTC0 : Outport  RequirementInfo={'linktype_rmi_doors' '000089b8 (/ESG Group/FDD Module Requirements/ES FDDs/CM475A - TSG31 Configuration and Use)' '#CM475A_58' 'true' 'REQ: CM475A_58' '' } %GIDa_a37e6da3_bb1e_40fb_821c_0bab706fa8f5
  RegOutpTSG31DTC1 : Outport  RequirementInfo={'linktype_rmi_doors' '000089b8 (/ESG Group/FDD Module Requirements/ES FDDs/CM475A - TSG31 Configuration and Use)' '#CM475A_58' 'true' 'REQ: CM475A_58' '' } %GIDa_f0a32233_38d5_4472_99b5_d78f5c529c5f  Port=2
  RegOutpTSG31CMP0E : Outport  Port=3
  RegOutpTSG31CMPUE : Outport  Port=4
  RegOutpTSG31CMPVE : Outport  Port=5
  RegOutpTSG31CMPWE : Outport  Port=6
  RegOutpTSG31DCMP0E : Outport  Port=7
  RegOutpTSG31CMP12E : Outport  Port=8
  RegOutpTSG31DCMP1E : Outport  Port=9
  RegOutpTSG31CMP7E : Outport  Port=10
  RegOutpTSG31CMP11E : Outport  Port=11
  wires:
  RawTime_NanoSec to RawTimerCount_Cnt Conversion Block1/1 -> Data Store Write/1, Subtract/2
  PWM Dead Band/1 -> RawTime_NanoSec to RawTimerCount_Cnt Conversion Block/1
  RawTime_NanoSec to RawTimerCount_Cnt Conversion Block/1 -> RegOutpTSG31DTC0/1, RegOutpTSG31DTC1/1
  Minimum PWM Period/1 -> RawTime_NanoSec to RawTimerCount_Cnt Conversion Block6/1
  PeakMtrCtrlADCOffset/1 -> RawTime_NanoSec to RawTimerCount_Cnt Conversion Block1/1
  MotAg0 SPI Transmission Start/1 -> RawTime_NanoSec to RawTimerCount_Cnt Conversion Block2/1
  RawTime_NanoSec to RawTimerCount_Cnt Conversion Block2/1 -> Data Store Write1/1, Subtract1/2
  2mSecADCOffset/1 -> RawTime_NanoSec to RawTimerCount_Cnt Conversion Block3/1
  VlyMtrCtrlADCOffset/1 -> RawTime_NanoSec to RawTimerCount_Cnt Conversion Block4/1
  TSG31UPDATE/1 -> RawTime_NanoSec to RawTimerCount_Cnt Conversion Block5/1
  RawTime_NanoSec to RawTimerCount_Cnt Conversion Block6/1 -> RegOutpTSG31CMPUE/1, RegOutpTSG31CMP0E/1, Subtract1/1, Subtract/1, RegOutpTSG31CMPWE/1, RegOutpTSG31CMPVE/1
  Subtract/1 -> Bitwise Operator1/1
  Bitwise Operator1/1 -> RegOutpTSG31DCMP0E/1
  Subtract1/1 -> Bitwise Operator2/1
  Bitwise Operator2/1 -> RegOutpTSG31CMP12E/1
  RawTime_NanoSec to RawTimerCount_Cnt Conversion Block3/1 -> Bitwise Operator3/1
  Bitwise Operator3/1 -> RegOutpTSG31DCMP1E/1
  RawTime_NanoSec to RawTimerCount_Cnt Conversion Block4/1 -> Bitwise Operator4/1
  Bitwise Operator4/1 -> RegOutpTSG31CMP7E/1
  RawTime_NanoSec to RawTimerCount_Cnt Conversion Block5/1 -> Bitwise Operator5/1
  Bitwise Operator5/1 -> RegOutpTSG31CMP11E/1

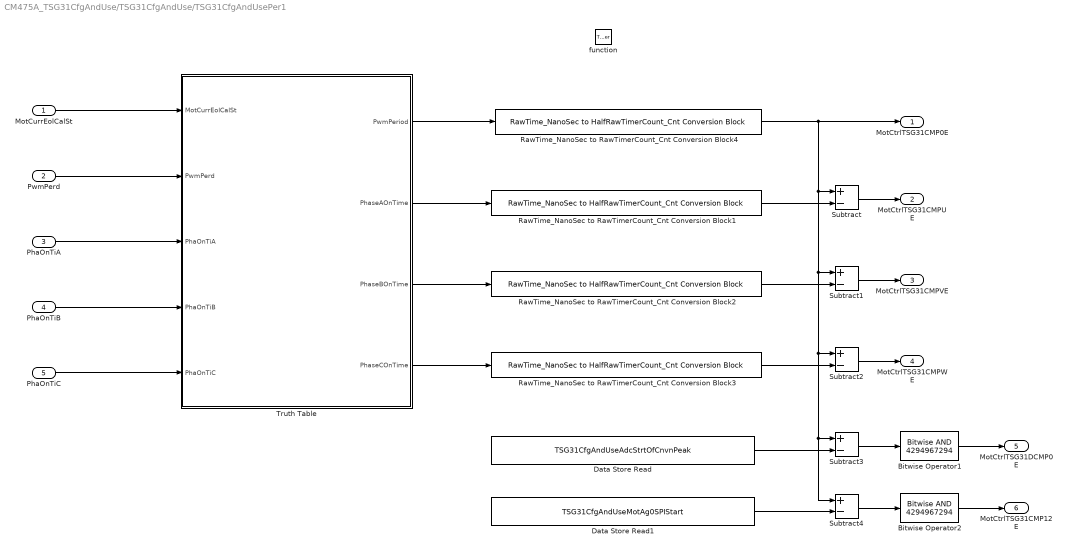
== system CM475A_TSG31CfgAndUse/TSG31CfgAndUse/TSG31CfgAndUsePer1 ==
  MotCurrEolCalSt : Inport
  PwmPerd : Inport  Port=2
  PhaOnTiA : Inport  Port=3
  PhaOnTiB : Inport  Port=4
  PhaOnTiC : Inport  Port=5
  function : TriggerPort  TriggerType=function-call
  Bitwise Operator1 : simulink/Logic and Bit Operations/Bitwise Operator  logicop=AND  UseBitMask=on  BitMask=4294967294  BitMaskRealWorld=Stored Integer
  Bitwise Operator2 : simulink/Logic and Bit Operations/Bitwise Operator  logicop=AND  UseBitMask=on  BitMask=4294967294  BitMaskRealWorld=Stored Integer
  Data Store Read : DataStoreRead  DataStoreName=TSG31CfgAndUseAdcStrtOfCnvnPeak
  Data Store Read1 : DataStoreRead  DataStoreName=TSG31CfgAndUseMotAg0SPIStart
  RawTime_NanoSec to RawTimerCount_Cnt Conversion Block{1..4} (4 alike) : CM475A_TSG31CfgAndUse_ModelLibrary_Rev001/RawTime_NanoSec to HalfRawTimerCount_Cnt Conversion Block
  Subtract{,1..4} (5 alike) : Sum  Inputs=+-
  Truth Table : Truth Table  TreatAsAtomicUnit=on
  MotCtrlTSG31CMP0E : Outport
  MotCtrlTSG31CMPUE : Outport  Port=2
  MotCtrlTSG31CMPVE : Outport  Port=3
  MotCtrlTSG31CMPWE : Outport  Port=4
  MotCtrlTSG31DCMP0E : Outport  Port=5
  MotCtrlTSG31CMP12E : Outport  Port=6
  wires:
  RawTime_NanoSec to RawTimerCount_Cnt Conversion Block1/1 -> Subtract/2
  Subtract/1 -> MotCtrlTSG31CMPUE/1
  Subtract1/1 -> MotCtrlTSG31CMPVE/1
  Subtract2/1 -> MotCtrlTSG31CMPWE/1
  Subtract3/1 -> Bitwise Operator1/1
  Subtract4/1 -> Bitwise Operator2/1
  RawTime_NanoSec to RawTimerCount_Cnt Conversion Block4/1 -> Subtract3/1, Subtract4/1, Subtract2/1, Subtract1/1, Subtract/1, MotCtrlTSG31CMP0E/1
  RawTime_NanoSec to RawTimerCount_Cnt Conversion Block2/1 -> Subtract1/2
  RawTime_NanoSec to RawTimerCount_Cnt Conversion Block3/1 -> Subtract2/2
  Data Store Read/1 -> Subtract3/2
  Data Store Read1/1 -> Subtract4/2
  MotCurrEolCalSt/1 -> Truth Table/1(MotCurrEolCalSt)
  Truth Table/1(PwmPeriod) -> RawTime_NanoSec to RawTimerCount_Cnt Conversion Block4/1
  Truth Table/2(PhaseAOnTime) -> RawTime_NanoSec to RawTimerCount_Cnt Conversion Block1/1
  Truth Table/3(PhaseBOnTime) -> RawTime_NanoSec to RawTimerCount_Cnt Conversion Block2/1
  Truth Table/4(PhaseCOnTime) -> RawTime_NanoSec to RawTimerCount_Cnt Conversion Block3/1
  PwmPerd/1 -> Truth Table/2(PwmPerd)
  PhaOnTiA/1 -> Truth Table/3(PhaOnTiA)
  PhaOnTiB/1 -> Truth Table/4(PhaOnTiB)
  PhaOnTiC/1 -> Truth Table/5(PhaOnTiC)
  Bitwise Operator1/1 -> MotCtrlTSG31DCMP0E/1
  Bitwise Operator2/1 -> MotCtrlTSG31CMP12E/1

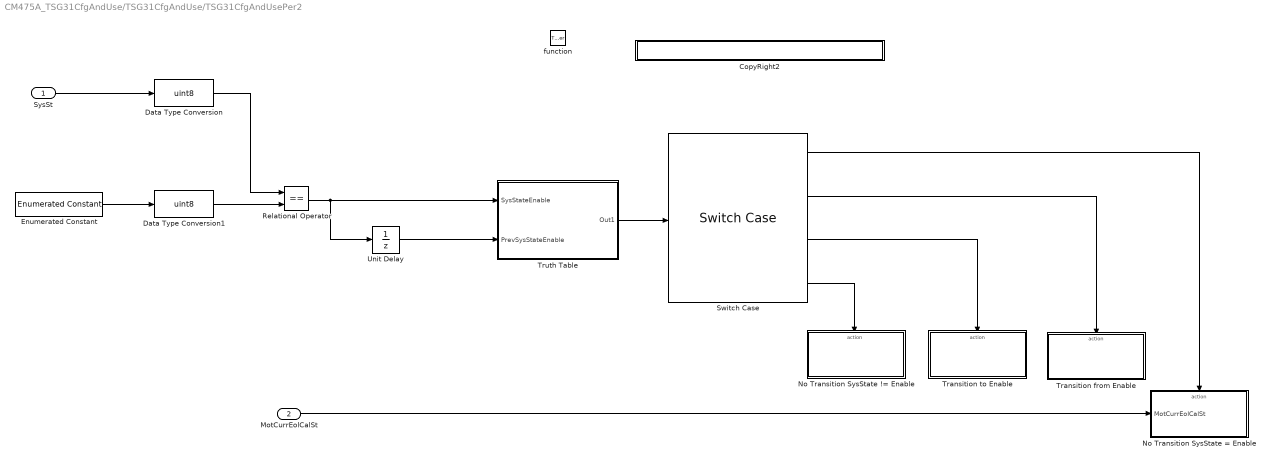
== system CM475A_TSG31CfgAndUse/TSG31CfgAndUse/TSG31CfgAndUsePer2 ==
  SysSt : Inport  OutDataTypeStr=Enum: SysSt1
  MotCurrEolCalSt : Inport  Port=2
  function : TriggerPort  TriggerType=function-call
  CopyRight2 : Subsystem  Description=|  mask(Copyright Information){none=on}
      | Copyright info block.                                               
      |                                                                     
      | Place copyright information at the top of every subsystem in design.
      mask prompts: none "No parameters"
      mask help: Place copyright information at the top of every subsystem in design.
      mask Display:
      | NxtrConf = 'Nexteer Confidential';
      | 
      | sys = bdroot; %handle for the current model ("system")
      | first = get_param(sys,'Created');
      | first = first(end-3:end);  %year is last four digits
      | 
      | last = get_param(sys,'LastModifiedDate');
      | if isempty(last)
      |     last = datestr(now,'yyyy');
      | else
      |     last = last(end-3:end);
      | end
      | 
      | if strcmp(first,last)
      |     fprintf('%s -- Copyright %s Nexteer',NxtrConf,first)
      | else
      |     fprintf('%s -- %s%s- %s Nexteer',NxtrConf,char(169),first,last)
      | end
  Data Type Conversion : DataTypeConversion  OutDataTypeStr=uint8
  Data Type Conversion1 : DataTypeConversion  OutDataTypeStr=uint8
  Enumerated Constant : simulink/Sources/Enumerated Constant  OutDataTypeStr=Enum: SysSt1  Value=SysSt1.SYSST_ENA  SampleTime=inf
  No Transition SysState != Enable : Subsystem  TreatAsAtomicUnit=on
  No Transition SysState = Enable : Subsystem  TreatAsAtomicUnit=on
  Relational Operator : RelationalOperator  Operator===  OutDataTypeStr=boolean
  Switch Case : SwitchCase  CaseConditions={1,2,3}
  Transition from Enable : Subsystem  TreatAsAtomicUnit=on
  Transition to Enable : Subsystem  TreatAsAtomicUnit=on
  Truth Table : Truth Table  TreatAsAtomicUnit=on
  Unit Delay : UnitDelay  SampleTime=-1  StateName=TSG31CfgAndUseSysStEnaPrev  StateMustResolveToSignalObject=on
      settings: AttributesFormatString=|
      | State Variable:
      | %<StateName>
  wires:
  Switch Case/1 -> No Transition SysState = Enable/Action
  Enumerated Constant/1 -> Data Type Conversion1/1
  Relational Operator/1 -> Unit Delay/1, Truth Table/1(SysStateEnable)
  Truth Table/1(Out1) -> Switch Case/1
  Switch Case/2 -> Transition from Enable/Action
  MotCurrEolCalSt/1 -> No Transition SysState = Enable/1(MotCurrEolCalSt)
  Switch Case/3 -> Transition to Enable/Action
  Switch Case/4 -> No Transition SysState != Enable/Action
  SysSt/1 -> Data Type Conversion/1
  Data Type Conversion1/1 -> Relational Operator/2
  Data Type Conversion/1 -> Relational Operator/1
  Unit Delay/1 -> Truth Table/2(PrevSysStateEnable)

== system CM475A_TSG31CfgAndUse/TSG31CfgAndUse/TSG31CfgAndUseInit1/CopyRight2 ==

== system CM475A_TSG31CfgAndUse/TSG31CfgAndUse/TSG31CfgAndUseInit1/Map FET Ctrl Signals to GPIO and Set Low ==
  CopyRight2 : Subsystem  Description=|  mask(Copyright Information){none=on}
      | Copyright info block.                                               
      |                                                                     
      | Place copyright information at the top of every subsystem in design.
      mask prompts: none "No parameters"
      mask help: Place copyright information at the top of every subsystem in design.
      mask Display:
      | NxtrConf = 'Nexteer Confidential';
      | 
      | sys = bdroot; %handle for the current model ("system")
      | first = get_param(sys,'Created');
      | first = first(end-3:end);  %year is last four digits
      | 
      | last = get_param(sys,'LastModifiedDate');
      | if isempty(last)
      |     last = datestr(now,'yyyy');
      | else
      |     last = last(end-3:end);
      | end
      | 
      | if strcmp(first,last)
      |     fprintf('%s -- Copyright %s Nexteer',NxtrConf,first)
      | else
      |     fprintf('%s -- %s%s- %s Nexteer',NxtrConf,char(169),first,last)
      | end
  Map Pins to GPIO : Subsystem  RequirementInfo={'linktype_rmi_doors' '000089b8 (/ESG Group/FDD Module Requirements/ES FDDs/CM475A - TSG31 Configuration and Use)' '#CM475A_15' 'true' 'REQ: CM475A_15' '' } %GIDa_309b5f00_7fe9_4a38_9d92_ce72005e381c  Priority=10  TreatAsAtomicUnit=on
      settings: AttributesFormatString=|
      | Priority:
      | %<Priority>
  Set GPIO Level : Subsystem  Priority=20  TreatAsAtomicUnit=on
      settings: AttributesFormatString=|
      | Priority:
      | %<Priority>

== system CM475A_TSG31CfgAndUse/TSG31CfgAndUse/TSG31CfgAndUsePer2/CopyRight2 ==

== system CM475A_TSG31CfgAndUse/TSG31CfgAndUse/TSG31CfgAndUsePer2/No Transition SysState != Enable ==
  note: Do Nothing
  Action Port : ActionPort  ActionType=default
  CopyRight2 : Subsystem  Description=|  mask(Copyright Information){none=on}
      | Copyright info block.                                               
      |                                                                     
      | Place copyright information at the top of every subsystem in design.
      mask prompts: none "No parameters"
      mask help: Place copyright information at the top of every subsystem in design.
      mask Display:
      | NxtrConf = 'Nexteer Confidential';
      | 
      | sys = bdroot; %handle for the current model ("system")
      | first = get_param(sys,'Created');
      | first = first(end-3:end);  %year is last four digits
      | 
      | last = get_param(sys,'LastModifiedDate');
      | if isempty(last)
      |     last = datestr(now,'yyyy');
      | else
      |     last = last(end-3:end);
      | end
      | 
      | if strcmp(first,last)
      |     fprintf('%s -- Copyright %s Nexteer',NxtrConf,first)
      | else
      |     fprintf('%s -- %s%s- %s Nexteer',NxtrConf,char(169),first,last)
      | end

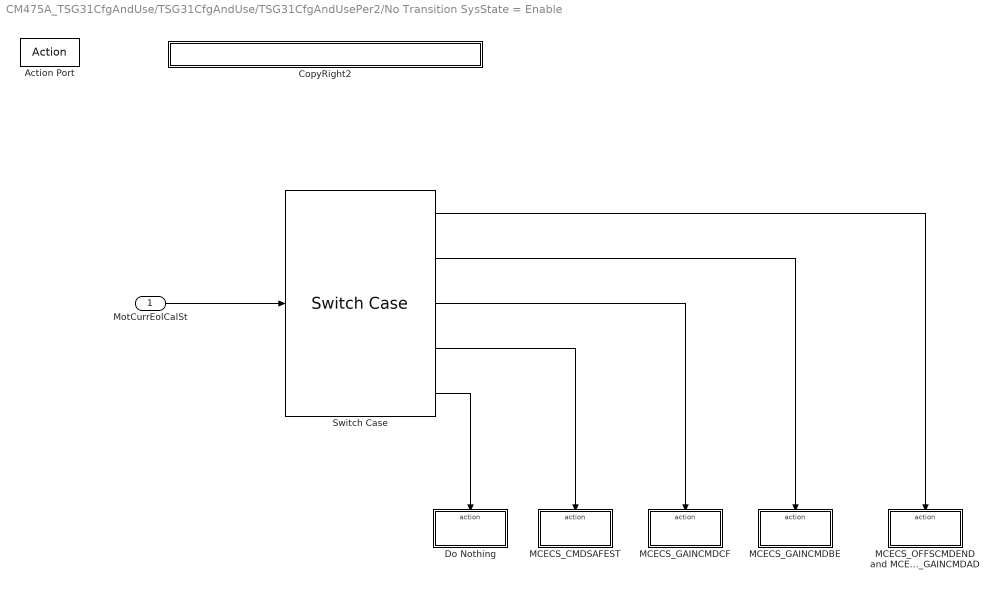
== system CM475A_TSG31CfgAndUse/TSG31CfgAndUse/TSG31CfgAndUsePer2/No Transition SysState = Enable ==
  MotCurrEolCalSt : Inport
  Action Port : ActionPort  ActionType=case
  CopyRight2 : Subsystem  Description=|  mask(Copyright Information){none=on}
      | Copyright info block.                                               
      |                                                                     
      | Place copyright information at the top of every subsystem in design.
      mask prompts: none "No parameters"
      mask help: Place copyright information at the top of every subsystem in design.
      mask Display:
      | NxtrConf = 'Nexteer Confidential';
      | 
      | sys = bdroot; %handle for the current model ("system")
      | first = get_param(sys,'Created');
      | first = first(end-3:end);  %year is last four digits
      | 
      | last = get_param(sys,'LastModifiedDate');
      | if isempty(last)
      |     last = datestr(now,'yyyy');
      | else
      |     last = last(end-3:end);
      | end
      | 
      | if strcmp(first,last)
      |     fprintf('%s -- Copyright %s Nexteer',NxtrConf,first)
      | else
      |     fprintf('%s -- %s%s- %s Nexteer',NxtrConf,char(169),first,last)
      | end
  Do Nothing : Subsystem  TreatAsAtomicUnit=on
  MCECS_CMDSAFEST : Subsystem  TreatAsAtomicUnit=on
  MCECS_GAINCMDBE : Subsystem  TreatAsAtomicUnit=on
  MCECS_GAINCMDCF : Subsystem  TreatAsAtomicUnit=on
  MCECS_OFFSCMDEND and MCECS_GAINCMDAD : Subsystem  TreatAsAtomicUnit=on
  Switch Case : SwitchCase  CaseConditions={[4,5],6,7,8}
  wires:
  MotCurrEolCalSt/1 -> Switch Case/1
  Switch Case/1 -> MCECS_OFFSCMDEND and MCECS_GAINCMDAD/Action
  Switch Case/2 -> MCECS_GAINCMDBE/Action
  Switch Case/3 -> MCECS_GAINCMDCF/Action
  Switch Case/4 -> MCECS_CMDSAFEST/Action
  Switch Case/5 -> Do Nothing/Action

== system CM475A_TSG31CfgAndUse/TSG31CfgAndUse/TSG31CfgAndUsePer2/Transition from Enable ==
  Action Port : ActionPort  ActionType=case
  CopyRight2 : Subsystem  Description=|  mask(Copyright Information){none=on}
      | Copyright info block.                                               
      |                                                                     
      | Place copyright information at the top of every subsystem in design.
      mask prompts: none "No parameters"
      mask help: Place copyright information at the top of every subsystem in design.
      mask Display:
      | NxtrConf = 'Nexteer Confidential';
      | 
      | sys = bdroot; %handle for the current model ("system")
      | first = get_param(sys,'Created');
      | first = first(end-3:end);  %year is last four digits
      | 
      | last = get_param(sys,'LastModifiedDate');
      | if isempty(last)
      |     last = datestr(now,'yyyy');
      | else
      |     last = last(end-3:end);
      | end
      | 
      | if strcmp(first,last)
      |     fprintf('%s -- Copyright %s Nexteer',NxtrConf,first)
      | else
      |     fprintf('%s -- %s%s- %s Nexteer',NxtrConf,char(169),first,last)
      | end
  Map FET Ctrl Signals to GPIO and Set Low : Subsystem  RequirementInfo={'linktype_rmi_doors' '000089b8 (/ESG Group/FDD Module Requirements/ES FDDs/CM475A - TSG31 Configuration and Use)' '#CM475A_15' 'true' 'REQ: CM475A_15' '' ; 'linktype_rmi_doors' '000089b8 (/ESG Group/FDD Module Requirements/ES FDDs/CM475A - TSG31 Configuration and Use)' '#CM475A_71' 'true' 'REQ: CM475A_71' '' ; 'linktype_rmi_doors' '000089b8 (/ESG Group/FDD Module Requirements/ES FDDs/CM475A - TSG31 Configuration and Use)' '#CM475A_70' 'true' 'REQ: CM475A_70' '' ; 'linktype_rmi_doors' '000089b8 (/ESG Group/FDD Module Requirements/ES FDDs/CM475A - TSG31 Configuration and Use)' '#CM475A_69' 'true' 'REQ: CM475A_69' '' ; 'linktype_rmi_doors' '000089b8 (/ESG Group/FDD Module Requirements/ES FDDs/CM475A - TSG31 Configuration and Use)' '#CM475A_68' 'true' 'REQ: CM475A_68' '' ; 'linktype_rmi_doors' '000089b8 (/ESG Group/FDD Module Requirements/ES FDDs/CM475A - TSG31 Configuration and Use)' '#CM475A_67' 'true' 'REQ: CM475A_67' '' } %GIDa_c907249a_7fd4_4784_bdee_42807a67f8dd

== system CM475A_TSG31CfgAndUse/TSG31CfgAndUse/TSG31CfgAndUsePer2/Transition to Enable ==
  Action Port : ActionPort  ActionType=case
  CopyRight2 : Subsystem  Description=|  mask(Copyright Information){none=on}
      | Copyright info block.                                               
      |                                                                     
      | Place copyright information at the top of every subsystem in design.
      mask prompts: none "No parameters"
      mask help: Place copyright information at the top of every subsystem in design.
      mask Display:
      | NxtrConf = 'Nexteer Confidential';
      | 
      | sys = bdroot; %handle for the current model ("system")
      | first = get_param(sys,'Created');
      | first = first(end-3:end);  %year is last four digits
      | 
      | last = get_param(sys,'LastModifiedDate');
      | if isempty(last)
      |     last = datestr(now,'yyyy');
      | else
      |     last = last(end-3:end);
      | end
      | 
      | if strcmp(first,last)
      |     fprintf('%s -- Copyright %s Nexteer',NxtrConf,first)
      | else
      |     fprintf('%s -- %s%s- %s Nexteer',NxtrConf,char(169),first,last)
      | end
  Map Pins to Peripheral : Subsystem  TreatAsAtomicUnit=on

== system CM475A_TSG31CfgAndUse/TSG31CfgAndUse/TSG31CfgAndUseInit1/Map FET Ctrl Signals to GPIO and Set Low/CopyRight2 ==

== system CM475A_TSG31CfgAndUse/TSG31CfgAndUse/TSG31CfgAndUseInit1/Map FET Ctrl Signals to GPIO and Set Low/Map Pins to GPIO ==
  CopyRight2 : Subsystem  Description=|  mask(Copyright Information){none=on}
      | Copyright info block.                                               
      |                                                                     
      | Place copyright information at the top of every subsystem in design.
      mask prompts: none "No parameters"
      mask help: Place copyright information at the top of every subsystem in design.
      mask Display:
      | NxtrConf = 'Nexteer Confidential';
      | 
      | sys = bdroot; %handle for the current model ("system")
      | first = get_param(sys,'Created');
      | first = first(end-3:end);  %year is last four digits
      | 
      | last = get_param(sys,'LastModifiedDate');
      | if isempty(last)
      |     last = datestr(now,'yyyy');
      | else
      |     last = last(end-3:end);
      | end
      | 
      | if strcmp(first,last)
      |     fprintf('%s -- Copyright %s Nexteer',NxtrConf,first)
      | else
      |     fprintf('%s -- %s%s- %s Nexteer',NxtrConf,char(169),first,last)
      | end
  IoHwAb_SetFctGpioPhaALowrCmd : Subsystem  TreatAsAtomicUnit=on
  IoHwAb_SetFctGpioPhaAUpprCmd : Subsystem  TreatAsAtomicUnit=on
  IoHwAb_SetFctGpioPhaBLowrCmd : Subsystem  TreatAsAtomicUnit=on
  IoHwAb_SetFctGpioPhaBUpprCmd : Subsystem  TreatAsAtomicUnit=on
  IoHwAb_SetFctGpioPhaCLowrCmd : Subsystem  TreatAsAtomicUnit=on
  IoHwAb_SetFctGpioPhaCUpprCmd : Subsystem  TreatAsAtomicUnit=on

== system CM475A_TSG31CfgAndUse/TSG31CfgAndUse/TSG31CfgAndUseInit1/Map FET Ctrl Signals to GPIO and Set Low/Set GPIO Level ==
  Constant : Constant  Value=0  OutDataTypeStr=boolean
  CopyRight2 : Subsystem  Description=|  mask(Copyright Information){none=on}
      | Copyright info block.                                               
      |                                                                     
      | Place copyright information at the top of every subsystem in design.
      mask prompts: none "No parameters"
      mask help: Place copyright information at the top of every subsystem in design.
      mask Display:
      | NxtrConf = 'Nexteer Confidential';
      | 
      | sys = bdroot; %handle for the current model ("system")
      | first = get_param(sys,'Created');
      | first = first(end-3:end);  %year is last four digits
      | 
      | last = get_param(sys,'LastModifiedDate');
      | if isempty(last)
      |     last = datestr(now,'yyyy');
      | else
      |     last = last(end-3:end);
      | end
      | 
      | if strcmp(first,last)
      |     fprintf('%s -- Copyright %s Nexteer',NxtrConf,first)
      | else
      |     fprintf('%s -- %s%s- %s Nexteer',NxtrConf,char(169),first,last)
      | end
  IoHwAb_SetGpioPhaALowrCmd : Subsystem  TreatAsAtomicUnit=on
  IoHwAb_SetGpioPhaAUpprCmd : Subsystem  TreatAsAtomicUnit=on
  IoHwAb_SetGpioPhaBLowrCmd : Subsystem  TreatAsAtomicUnit=on
  IoHwAb_SetGpioPhaBUpprCmd : Subsystem  TreatAsAtomicUnit=on
  IoHwAb_SetGpioPhaCLowrCmd : Subsystem  TreatAsAtomicUnit=on
  IoHwAb_SetGpioPhaCUpprCmd : Subsystem  TreatAsAtomicUnit=on
  wires:
  Constant/1 -> IoHwAb_SetGpioPhaALowrCmd/1(PinSt), IoHwAb_SetGpioPhaCUpprCmd/1(PinSt), IoHwAb_SetGpioPhaBUpprCmd/1(PinSt), IoHwAb_SetGpioPhaAUpprCmd/1(PinSt), IoHwAb_SetGpioPhaCLowrCmd/1(PinSt), IoHwAb_SetGpioPhaBLowrCmd/1(PinSt)

== system CM475A_TSG31CfgAndUse/TSG31CfgAndUse/TSG31CfgAndUsePer2/No Transition SysState != Enable/CopyRight2 ==

== system CM475A_TSG31CfgAndUse/TSG31CfgAndUse/TSG31CfgAndUsePer2/No Transition SysState = Enable/CopyRight2 ==

== system CM475A_TSG31CfgAndUse/TSG31CfgAndUse/TSG31CfgAndUsePer2/No Transition SysState = Enable/Do Nothing ==
  note: Do Nothing
  Action Port : ActionPort  ActionType=default
  CopyRight2 : Subsystem  Description=|  mask(Copyright Information){none=on}
      | Copyright info block.                                               
      |                                                                     
      | Place copyright information at the top of every subsystem in design.
      mask prompts: none "No parameters"
      mask help: Place copyright information at the top of every subsystem in design.
      mask Display:
      | NxtrConf = 'Nexteer Confidential';
      | 
      | sys = bdroot; %handle for the current model ("system")
      | first = get_param(sys,'Created');
      | first = first(end-3:end);  %year is last four digits
      | 
      | last = get_param(sys,'LastModifiedDate');
      | if isempty(last)
      |     last = datestr(now,'yyyy');
      | else
      |     last = last(end-3:end);
      | end
      | 
      | if strcmp(first,last)
      |     fprintf('%s -- Copyright %s Nexteer',NxtrConf,first)
      | else
      |     fprintf('%s -- %s%s- %s Nexteer',NxtrConf,char(169),first,last)
      | end

== system CM475A_TSG31CfgAndUse/TSG31CfgAndUse/TSG31CfgAndUsePer2/No Transition SysState = Enable/MCECS_CMDSAFEST ==
  Action Port : ActionPort  ActionType=case
  CopyRight2 : Subsystem  Description=|  mask(Copyright Information){none=on}
      | Copyright info block.                                               
      |                                                                     
      | Place copyright information at the top of every subsystem in design.
      mask prompts: none "No parameters"
      mask help: Place copyright information at the top of every subsystem in design.
      mask Display:
      | NxtrConf = 'Nexteer Confidential';
      | 
      | sys = bdroot; %handle for the current model ("system")
      | first = get_param(sys,'Created');
      | first = first(end-3:end);  %year is last four digits
      | 
      | last = get_param(sys,'LastModifiedDate');
      | if isempty(last)
      |     last = datestr(now,'yyyy');
      | else
      |     last = last(end-3:end);
      | end
      | 
      | if strcmp(first,last)
      |     fprintf('%s -- Copyright %s Nexteer',NxtrConf,first)
      | else
      |     fprintf('%s -- %s%s- %s Nexteer',NxtrConf,char(169),first,last)
      | end
  Map Pins to GPIO : Subsystem  Priority=10  TreatAsAtomicUnit=on
      settings: AttributesFormatString=|
      | Priority:
      | %<Priority>
  Set GPIO Level : Subsystem  Priority=20  TreatAsAtomicUnit=on
      settings: AttributesFormatString=|
      | Priority:
      | %<Priority>

== system CM475A_TSG31CfgAndUse/TSG31CfgAndUse/TSG31CfgAndUsePer2/No Transition SysState = Enable/MCECS_GAINCMDBE ==
  Action Port : ActionPort  ActionType=case
  CopyRight2 : Subsystem  Description=|  mask(Copyright Information){none=on}
      | Copyright info block.                                               
      |                                                                     
      | Place copyright information at the top of every subsystem in design.
      mask prompts: none "No parameters"
      mask help: Place copyright information at the top of every subsystem in design.
      mask Display:
      | NxtrConf = 'Nexteer Confidential';
      | 
      | sys = bdroot; %handle for the current model ("system")
      | first = get_param(sys,'Created');
      | first = first(end-3:end);  %year is last four digits
      | 
      | last = get_param(sys,'LastModifiedDate');
      | if isempty(last)
      |     last = datestr(now,'yyyy');
      | else
      |     last = last(end-3:end);
      | end
      | 
      | if strcmp(first,last)
      |     fprintf('%s -- Copyright %s Nexteer',NxtrConf,first)
      | else
      |     fprintf('%s -- %s%s- %s Nexteer',NxtrConf,char(169),first,last)
      | end
  Map Pins to GPIO : Subsystem  Priority=10  TreatAsAtomicUnit=on
      settings: AttributesFormatString=|
      | Priority:
      | %<Priority>
  Set GPIO Level : Subsystem  Priority=20  TreatAsAtomicUnit=on
      settings: AttributesFormatString=|
      | Priority:
      | %<Priority>
